simulink model "Labo4_Simulink"  (R2024a)
settings: Solver=ode45  StartTime=0.0  StopTime=0.02  MaxStep=1e-5  RelTol=1e-3
settings Model: Creator=alexande.seite  LastModifiedBy=alexande.seite

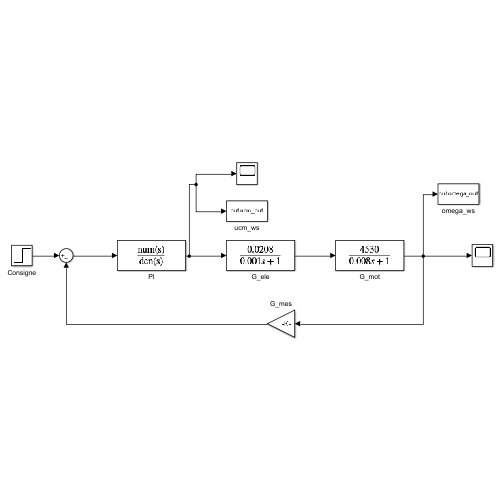
[thumbnail: Simulink's stored preview of the top-level diagram]
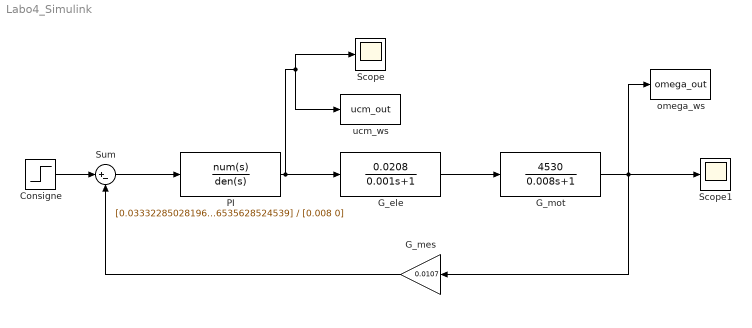
== system Labo4_Simulink ==
  Consigne : Step  Time=0  After=0.107  SampleTime=0
  G_ele : TransferFcn  Numerator=0.0208  Denominator=[0.001 1]
  G_mes : Gain  Gain=0.0107
  G_mot : TransferFcn  Numerator=4530  Denominator=[0.008 1]
  PI : TransferFcn  Numerator=[0.0333228502819631 4.16535628524539]  Denominator=[0.008 0]
  Scope : Scope
  Scope1 : Scope
  Sum : Sum  Inputs=|+-
  omega_ws : ToWorkspace  VariableName=omega_out  SaveFormat=Structure With Time  SampleTime=-1
  ucm_ws : ToWorkspace  VariableName=ucm_out  SaveFormat=Structure With Time  SampleTime=-1
  wires:
  Sum/1 -> PI/1
  PI/1 -> Scope/1, ucm_ws/1, G_ele/1
  G_ele/1 -> G_mot/1
  G_mot/1 -> G_mes/1, omega_ws/1, Scope1/1
  Consigne/1 -> Sum/1
  G_mes/1 -> Sum/2
